simulink model "Hybrid_Beamforming"  (R2022b)
settings: Solver=FixedStepDiscrete  StartTime=0.0  StopTime=10  RelTol=1e-3
PreLoadFcn:
  | helperslexHybridBeamformingParam;
undefined symbols (not defined in the file or in its folder): paramHybridBF
libraries: dspmtrx3 x5, simulink x2, commrandsrc3 x1, phasedtxrxlib x1, commdigbbndam3 x1
CloseFcn:
  | clear paramHybridBF;
settings Model: FPTRunName=Active  ModifiedByFormat=The MathWorks Inc.  SimulationMode=accelerator  Creator=The MathWorks, Inc.  LastModifiedBy=The MathWorks Inc.
settings SolverCC: AlgebraicLoopSolver=TrustRegion  MaxZcPerStep=1
settings DataIOCC: LimitDataPoints=on  SaveFormat=Structure  SaveOutput=off  DSMLogging=off  SaveTime=off  ReturnWorkspaceOutputs=off
settings OptimizationCC: BlockReduction=off  ConditionallyExecuteInputs=off  DefaultParameterBehavior=Inlined  ExpressionDepthLimit=2147483647  LocalBlockOutputs=off  EfficientMapNaN2IntZero=off  LifeSpan=inf  SimCompilerOptimization=on
settings DebuggingCC: AlgebraicLoopMsg=error  UnderspecifiedInitializationDetection=Classic  MergeDetectMultiDrivingBlocksExec=none  SolverPrmCheckMsg=warning  MultiTaskDSMMsg=warning  MultiTaskCondExecSysMsg=none  SingleTaskRateTransMsg=error  IntegerOverflowMsg=none  ParameterPrecisionLossMsg=none  FcnCallInpInsideContextMsg=warning  UnconnectedInputMsg=warning  UnconnectedOutputMsg=warning  UnconnectedLineMsg=warning  AllowSymbolicDim=off  StateNameClashWarn=warning  PregeneratedLibrarySubsystemCodeDiagnostic=none  SFUnexpectedBacktrackingDiag=warning  SFNoUnconditionalDefaultTransitionDiag=warning  SFExecutionAtInitializationDiag=none  SFMachineParentedDataDiag=warning  ArithmeticOperatorsInVariantConditions=warning
settings HardwareCC: ProdBitPerPointer=32  ProdBitPerSizeT=32  ProdBitPerPtrDiffT=32  ProdLargestAtomicFloat=None  ProdIntDivRoundTo=Undefined  ProdEndianess=Unspecified  ProdWordSize=32  ProdHWDeviceType=ASIC/FPGA->ASIC/FPGA  TargetBitPerPointer=64  TargetBitPerSizeT=64  TargetBitPerPtrDiffT=64  TargetLongLongMode=on  TargetIntDivRoundTo=Zero  TargetEndianess=LittleEndian  TargetWordSize=64  TargetHWDeviceType=MATLAB Host  ProdEqTarget=off
settings ModelReferenceCC: EnableRefExpFcnMdlSchedulingChecks=on  PropagateSignalLabelsOutOfModel=off
settings SFSimCC: SimUseLocalCustomCode=off  CustomCodeUndefinedFunction=UseInterfaceOnly
settings RTWCC: DLArmComputeVersion=19.05
settings CodeAppCC: MaxIdLength=128
settings GRTTargetCC: TargetLangStandard=C89/C90 (ANSI)  CombineOutputUpdateFcns=off  GRTInterface=on
settings ConfigComp: CovMetricSettings=dw  CovSaveCumulativeToWorkspaceVar=on  CovSaveSingleToWorkspaceVar=on  CovExternalEMLEnable=off  CovSFcnEnable=off

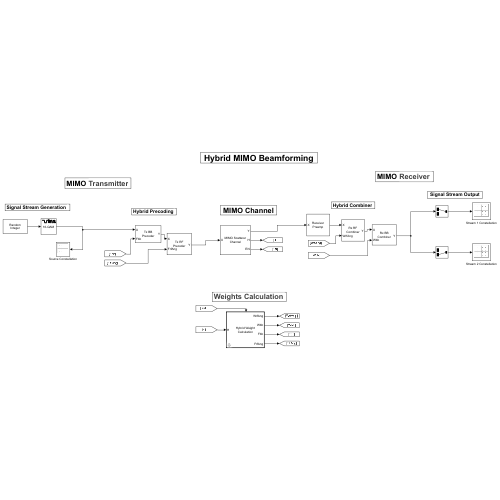
[thumbnail: Simulink's stored preview of the top-level diagram]
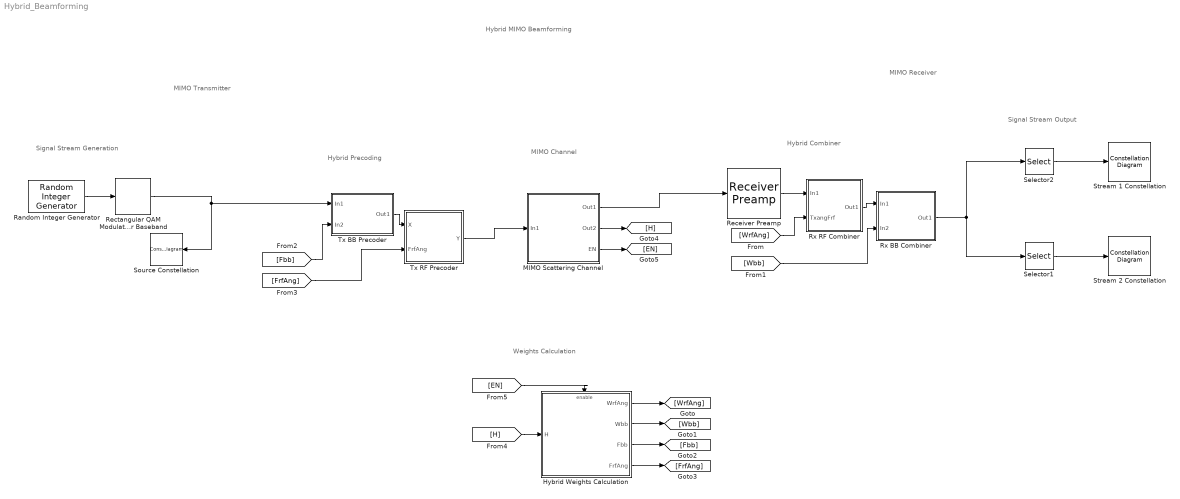
== system Hybrid_Beamforming ==
  note: Hybrid MIMO Beamforming
  note: Signal Stream Generation
  note: Hybrid Precoding
  note: MIMO Channel
  note: Signal Stream Output
  note: Hybrid Combiner
  note: Weights Calculation
  note: MIMO Transmitter
  note: MIMO Receiver
  Hybrid Weights Calculation : Subsystem  mask(Hybrid Beamforming Weights){Algorithm=QSHB, Ns=paramHybridBF.Ns, txpos=paramHybridBF.TxPos, NtRF=paramHybridBF.NtRF, rxpos=paramHybridBF.RxPos, NrRF=paramHybridBF.NrRF, txangF=paramHybridBF.TxAngF, rxangW=paramHybridBF.RxAngW, noisevar=1/paramHybridBF.SNR}
      mask prompts: Ns "Number of Data Streams"; txpos "Transmit Antenna Position"; NtRF "Number of Transmit RF Chain"; rxpos "Receive Antenna Position"; NrRF "Number of Receive RF Chain"; txangF "Transmit Direction Grid"; rxangW "Receive Direction Grid"; noisevar "Noise Power"
      mask help: Compute precoding and combining weights based on MIMO channel matrix
      mask init:
      | if strcmp(Algorithm,'QSHB')
      |     WSEL = 1;
      | else
      |     WSEL = 0;
      | end
      mask TypeOptions Algorithm: QSHB | HBPS
      mask Display:
      | disp('Hybrid Weight\nCalculation');
      | port_label('input',1,'H');
      | port_label('output',1,'WrfAng');
      | port_label('output',2,'Wbb');
      | port_label('output',3,'Fbb');
      | port_label('output',4,'FrfAng');
  MIMO Scattering Channel : Subsystem
      mask Display:
      | disp('MIMO Scatterer\nChannel');
      | port_label('input',1,'X');
      | port_label('output',1,'Y');
      | port_label('output',2,'H');
      | port_label('output',3,'EN');
  Random Integer Generator : commrandsrc3/Random Integer Generator  SetSize=paramHybridBF.M  SeedSource=Parameter  Seed=109  SampleTime=0.001  SamplesPerFrame=paramHybridBF.Ns  OutputDataType=double  SimulateUsing=Interpreted execution
  Receiver Preamp : phasedtxrxlib/Receiver Preamp  Gain=0  LossFactor=0  NoiseMethod=Noise power  NoiseFigure=0  ReferenceTemperature=290  SampleRateFromInputCheckbox=on  SampleRate=1e6  NoisePower=paramHybridBF.Ns/paramHybridBF.SNR  EnableInputPort=off  PhaseNoiseInputPort=off  SeedSource=Property  Seed=randi(65535,1)  SimulateUsing=Interpreted execution
  Rectangular QAM Modulator Baseband : commdigbbndam3/Rectangular QAM Modulator Baseband  M=paramHybridBF.M  InType=Integer  Enc=Gray  Mapping=[0:15]  PowType=Min. distance between symbols  MinDist=2/3  AvgPow=1  PeakPow=1  Ph=0  outDtype=double  outWordLen=16  outUDDataType=sfix(16)  outFracLenMode=Best precision  outFracLen=15  outDataTypeStr=double  outLastDataTypeStr=double
  Rx BB Combiner : Subsystem
      mask Display:
      | disp('Rx BB\nCombiner');
      | port_label('input',1,'X');
      | port_label('input',2,'Wbb');
      | port_label('output',1,'Y');
  Rx RF Combiner : Subsystem
      mask Display:
      | disp('Rx RF\nCombiner');
      | port_label('input',1,'X');
      | port_label('input',2,'WrfAng');
      | port_label('output',1,'Y');
  Selector1 : Selector  InputPortWidth=paramHybridBF.Ns  IndexOptions=Index vector (dialog)  Indices=2  OutputSizes=1
  Selector2 : Selector  InputPortWidth=paramHybridBF.Ns  IndexOptions=Index vector (dialog)  Indices=[1]  OutputSizes=1
  Source Constellation : ConstellationDiagram  WindowPosition=[298.000000,334.000000,438.000000,299.000000,]  ScopeFrameLocation=window  SymbolsToDisplaySource=Property  SymbolsToDisplay=paramHybridBF.NTxSym  ReferenceConstellation={[-10 -10]}  XLimits=[-2 2]  YLimits=[-2 2]  ShowReferenceConstellation=off  DefaultConfigurationName=comm.scopes.ConstellationDiagramBlockCfg
  Stream 1 Constellation : ConstellationDiagram  WindowPosition=[755.000000,331.000000,440.000000,303.000000,]  ScopeFrameLocation=window  SymbolsToDisplaySource=Property  SymbolsToDisplay=1000  ReferenceConstellation="{[-1+1i              -1+0.33333i              -1-0.33333i                    -1-1i              -0.33333+1i        -0.33333+0.33333i        -0.33333-0.33333i              -0.33333-1i               0.33333+1i         0.33333+0.33333i         0.33333-0.33333i               0.33333-1i                     1+1i               1+0.33333i               1-0.33333i                     1-1i]}"  XLimits=[-2 2]  YLimits=[-2 2]  DefaultConfigurationName=comm.scopes.ConstellationDiagramBlockCfg
  Stream 2 Constellation : ConstellationDiagram  WindowPosition=[788.000000,213.000000,485.000000,463.000000,]  ScopeFrameLocation=window  SymbolsToDisplaySource=Property  SymbolsToDisplay=1000  ReferenceConstellation="{[-1+1i              -1+0.33333i              -1-0.33333i                    -1-1i              -0.33333+1i        -0.33333+0.33333i        -0.33333-0.33333i              -0.33333-1i               0.33333+1i         0.33333+0.33333i         0.33333-0.33333i               0.33333-1i                     1+1i               1+0.33333i               1-0.33333i                     1-1i]}"  XLimits=[-2 2]  YLimits=[-2 2]  DefaultConfigurationName=comm.scopes.ConstellationDiagramBlockCfg
  Tx BB Precoder : Subsystem
      mask Display:
      | disp('Tx BB\nPrecoder');
      | port_label('input',1,'X');
      | port_label('Output',1,'Y');
      | port_label('Input',2,'Fbb');
  Tx RF Precoder : Subsystem
      mask Display:
      | disp('Tx RF\nPrecoder');
      | port_label('input',1,'X');
      | port_label('input',2,'FrfAng');
      | port_label('output',1,'Y');
  wires:
  Rx RF Combiner/1(Out1) -> Rx BB Combiner/1(In1)
  Rx BB Combiner/1(Out1) -> Selector2/1, Selector1/1
  Tx BB Precoder/1(Out1) -> Tx RF Precoder/1(X)
  Random Integer Generator/1 -> Rectangular QAM Modulator Baseband/1
  Rectangular QAM Modulator Baseband/1 -> Tx BB Precoder/1(In1), Source Constellation/1
  Selector1/1 -> Stream 2 Constellation/1
  Selector2/1 -> Stream 1 Constellation/1
  Tx RF Precoder/1(Y) -> MIMO Scattering Channel/1(In1)
  Hybrid Weights Calculation/1(WrfAng) -> [WrfAng]
  [WrfAng] -> Rx RF Combiner/2(TxangFrf)
  Hybrid Weights Calculation/2(Wbb) -> [Wbb]
  [Wbb] -> Rx BB Combiner/2(In2)
  Hybrid Weights Calculation/3(Fbb) -> [Fbb]
  [Fbb] -> Tx BB Precoder/2(In2)
  Hybrid Weights Calculation/4(FrfAng) -> [FrfAng]
  [FrfAng] -> Tx RF Precoder/2(FrfAng)
  MIMO Scattering Channel/2(Out2) -> [H]
  [H] -> Hybrid Weights Calculation/1(H)
  MIMO Scattering Channel/3(EN) -> [EN]
  [EN] -> Hybrid Weights Calculation/Enable
  MIMO Scattering Channel/1(Out1) -> Receiver Preamp/1
  Receiver Preamp/1 -> Rx RF Combiner/1(In1)

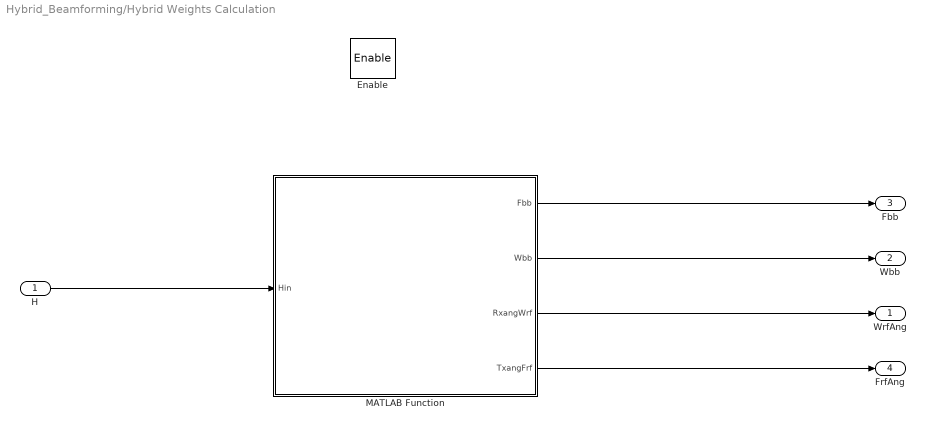
== system Hybrid_Beamforming/Hybrid Weights Calculation ==
  H : Inport
  Enable : EnablePort  PropagateVarSize=During execution
  MATLAB Function : MATLAB Function  TreatAsAtomicUnit=on
  WrfAng : Outport  VectorParamsAs1DForOutWhenUnconnected=off
  Wbb : Outport  Port=2  VectorParamsAs1DForOutWhenUnconnected=off
  Fbb : Outport  Port=3  VectorParamsAs1DForOutWhenUnconnected=off
  FrfAng : Outport  Port=4  VectorParamsAs1DForOutWhenUnconnected=off
  wires:
  H/1 -> MATLAB Function/1(Hin)
  MATLAB Function/1(Fbb) -> Fbb/1
  MATLAB Function/4(TxangFrf) -> FrfAng/1
  MATLAB Function/2(Wbb) -> Wbb/1
  MATLAB Function/3(RxangWrf) -> WrfAng/1

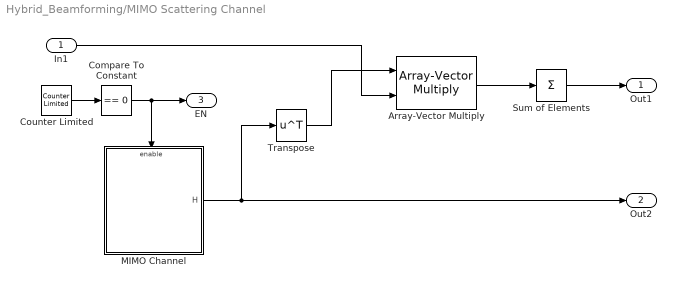
== system Hybrid_Beamforming/MIMO Scattering Channel ==
  In1 : Inport
  Array-Vector Multiply : dspmtrx3/Array-Vector Multiply  mode=Mute  saveAsFlag=0  Dimension=2  V_Source=Input port  V_VectFromMask=[0.5 0.25]  roundingMode=Floor  overflowMode=off  firstCoeffSignedness=Auto  firstCoeffDataTypeStr=Inherit: Same word length as input  firstCoeffMin=[]  firstCoeffMax=[]  firstCoeffLastDataTypeStr=Inherit: Same word length as input  prodOutputSignedness=Auto  accumSignedness=Auto  outputSignedness=Auto  outputDataTypeStr=Inherit: Same as product output  outputMin=[]  outputMax=[]  outputLastDataTypeStr=Inherit: Same as product output
  Compare To Constant : simulink/Logic and Bit Operations/Compare To Constant  relop===  const=0  OutDataTypeStr=boolean
  Counter Limited : simulink/Sources/Counter Limited  uplimit=paramHybridBF.NTxSym  tsamp=-1
  MIMO Channel : Subsystem
      mask Display:
      | disp('Channel')
      | port_label('output',1,'H')
      | port_label('input',1,'En')
  Sum of Elements : Sum  Inputs=+  CollapseMode=Specified dimension  CollapseDim=2
  Transpose : Math  Operator=transpose  SignedPower=on
  Out1 : Outport  VectorParamsAs1DForOutWhenUnconnected=off
  Out2 : Outport  Port=2  VectorParamsAs1DForOutWhenUnconnected=off
  EN : Outport  Port=3  VectorParamsAs1DForOutWhenUnconnected=off
  wires:
  Transpose/1 -> Array-Vector Multiply/1
  Compare To Constant/1 -> EN/1, MIMO Channel/Enable
  Counter Limited/1 -> Compare To Constant/1
  MIMO Channel/1(H) -> Transpose/1, Out2/1
  Array-Vector Multiply/1 -> Sum of Elements/1
  In1/1 -> Array-Vector Multiply/2
  Sum of Elements/1 -> Out1/1

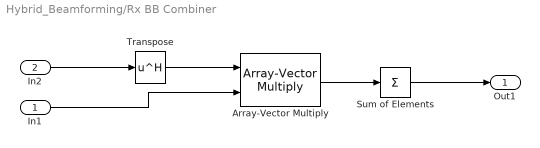
== system Hybrid_Beamforming/Rx BB Combiner ==
  In1 : Inport
  In2 : Inport  Port=2
  Array-Vector Multiply : dspmtrx3/Array-Vector Multiply  mode=Mute  saveAsFlag=0  Dimension=paramHybridBF.Ns  V_Source=Input port  V_VectFromMask=[0.5 0.25]  roundingMode=Floor  overflowMode=off  firstCoeffSignedness=Auto  firstCoeffDataTypeStr=Inherit: Same word length as input  firstCoeffMin=[]  firstCoeffMax=[]  firstCoeffLastDataTypeStr=Inherit: Same word length as input  prodOutputSignedness=Auto  accumSignedness=Auto  outputSignedness=Auto  outputDataTypeStr=Inherit: Same as product output  outputMin=[]  outputMax=[]  outputLastDataTypeStr=Inherit: Same as product output
  Sum of Elements : Sum  Inputs=+  CollapseMode=Specified dimension  CollapseDim=2
  Transpose : Math  Operator=hermitian  SignedPower=on
  Out1 : Outport  VectorParamsAs1DForOutWhenUnconnected=off
  wires:
  Array-Vector Multiply/1 -> Sum of Elements/1
  In2/1 -> Transpose/1
  Sum of Elements/1 -> Out1/1
  Transpose/1 -> Array-Vector Multiply/1
  In1/1 -> Array-Vector Multiply/2

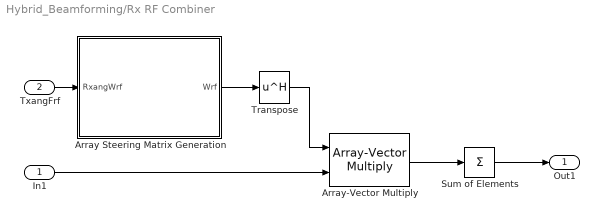
== system Hybrid_Beamforming/Rx RF Combiner ==
  In1 : Inport
  TxangFrf : Inport  Port=2
  Array Steering Matrix Generation : MATLAB Function  TreatAsAtomicUnit=on  mask(Steering Vector){RxPos=paramHybridBF.RxPos}
      mask prompts: RxPos "Receive Antenna Position"
      mask help: Compute array steering vector
  Array-Vector Multiply : dspmtrx3/Array-Vector Multiply  mode=Mute  saveAsFlag=0  Dimension=2  V_Source=Input port  V_VectFromMask=[0.5 0.25]  roundingMode=Floor  overflowMode=off  firstCoeffSignedness=Auto  firstCoeffDataTypeStr=Inherit: Same word length as input  firstCoeffMin=[]  firstCoeffMax=[]  firstCoeffLastDataTypeStr=Inherit: Same word length as input  prodOutputSignedness=Auto  accumSignedness=Auto  outputSignedness=Auto  outputDataTypeStr=Inherit: Same as product output  outputMin=[]  outputMax=[]  outputLastDataTypeStr=Inherit: Same as product output
  Sum of Elements : Sum  Inputs=+  CollapseMode=Specified dimension  CollapseDim=2
  Transpose : Math  Operator=hermitian  SignedPower=on
  Out1 : Outport  VectorParamsAs1DForOutWhenUnconnected=off
  wires:
  Array-Vector Multiply/1 -> Sum of Elements/1
  In1/1 -> Array-Vector Multiply/2
  Sum of Elements/1 -> Out1/1
  Transpose/1 -> Array-Vector Multiply/1
  TxangFrf/1 -> Array Steering Matrix Generation/1(RxangWrf)
  Array Steering Matrix Generation/1(Wrf) -> Transpose/1

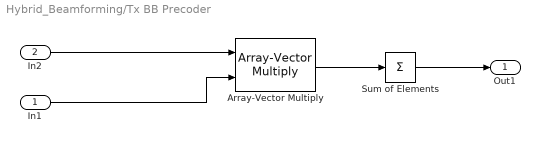
== system Hybrid_Beamforming/Tx BB Precoder ==
  In1 : Inport
  In2 : Inport  Port=2
  Array-Vector Multiply : dspmtrx3/Array-Vector Multiply  mode=Mute  saveAsFlag=0  Dimension=2  V_Source=Input port  V_VectFromMask=[0.5 0.25]  roundingMode=Floor  overflowMode=off  firstCoeffSignedness=Auto  firstCoeffDataTypeStr=Inherit: Same word length as input  firstCoeffMin=[]  firstCoeffMax=[]  firstCoeffLastDataTypeStr=Inherit: Same word length as input  prodOutputSignedness=Auto  accumSignedness=Auto  outputSignedness=Auto  outputDataTypeStr=Inherit: Same as product output  outputMin=[]  outputMax=[]  outputLastDataTypeStr=Inherit: Same as product output
  Sum of Elements : Sum  Inputs=+  CollapseMode=Specified dimension  CollapseDim=2
  Out1 : Outport  VectorParamsAs1DForOutWhenUnconnected=off
  wires:
  In2/1 -> Array-Vector Multiply/1
  In1/1 -> Array-Vector Multiply/2
  Array-Vector Multiply/1 -> Sum of Elements/1
  Sum of Elements/1 -> Out1/1

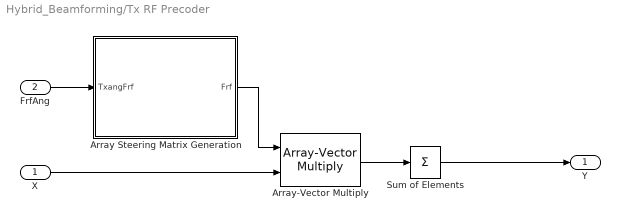
== system Hybrid_Beamforming/Tx RF Precoder ==
  X : Inport
  FrfAng : Inport  Port=2
  Array Steering Matrix Generation : MATLAB Function  TreatAsAtomicUnit=on  mask(Steering Vector){TxPos=paramHybridBF.TxPos}
      mask prompts: TxPos "Transmit Antenna Position"
      mask help: Compute array steering vector
  Array-Vector Multiply : dspmtrx3/Array-Vector Multiply  mode=Mute  saveAsFlag=0  Dimension=2  V_Source=Input port  V_VectFromMask=[0.5 0.25]  roundingMode=Floor  overflowMode=off  firstCoeffSignedness=Auto  firstCoeffDataTypeStr=Inherit: Same word length as input  firstCoeffMin=[]  firstCoeffMax=[]  firstCoeffLastDataTypeStr=Inherit: Same word length as input  prodOutputSignedness=Auto  accumSignedness=Auto  outputSignedness=Auto  outputDataTypeStr=Inherit: Same as product output  outputMin=[]  outputMax=[]  outputLastDataTypeStr=Inherit: Same as product output
  Sum of Elements : Sum  Inputs=+  CollapseMode=Specified dimension  CollapseDim=2
  Y : Outport  VectorParamsAs1DForOutWhenUnconnected=off
  wires:
  X/1 -> Array-Vector Multiply/2
  FrfAng/1 -> Array Steering Matrix Generation/1(TxangFrf)
  Array-Vector Multiply/1 -> Sum of Elements/1
  Sum of Elements/1 -> Y/1
  Array Steering Matrix Generation/1(Frf) -> Array-Vector Multiply/1

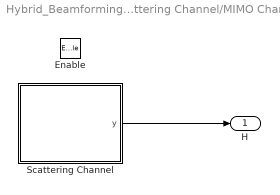
== system Hybrid_Beamforming/MIMO Scattering Channel/MIMO Channel ==
  Enable : EnablePort  PropagateVarSize=During execution
  "Scattering Channel " : MATLAB Function  TreatAsAtomicUnit=on  mask(MIMO Scattering Channel){txpos=paramHybridBF.TxPos, rxpos=paramHybridBF.RxPos}
      mask prompts: txpos "Tx Array Element Position"; rxpos "Rx Array Element Position"
      mask help: Create MIMO scattering channel matrix
  H : Outport  VectorParamsAs1DForOutWhenUnconnected=off
  wires:
  "Scattering Channel "/1(y) -> H/1

== matlab function Hybrid_Beamforming/Rx RF Combiner/Array Steering Matrix Generation ==
  data: RxangWrf input; Wrf output; RxPos parameter
function Wrf = fsteering_rx(RxangWrf,RxPos)
% Nr = size(RxPos,2);
% aa=ones(2,NrRF);
% arr=complex(zeros(Nr,NrRF));
% aa(:,1:NrRF)=RxangWrf(:,1:NrRF);
% 
% for i=1:NrRF
%     ang=aa(:,i);
%     arr(:,i)=steervec(RxPos,ang(:,1));
% end
% 
% Wrf = arr;

Wrf = steervec(RxPos,RxangWrf);

== matlab function Hybrid_Beamforming/Hybrid Weights Calculation/MATLAB Function ==
  data: Hin input; Fbb output; Wbb output; RxangWrf output; NtRF parameter; NrRF parameter; Ns parameter; txangF parameter; rxangW parameter; txpos parameter; rxpos parameter; noisevar parameter; Algorithm parameter; TxangFrf output
function [Fbb,Wbb, RxangWrf, TxangFrf] = hybridbfweights(Hin,NtRF, NrRF, Ns, txangF, rxangW, txpos, rxpos, noisevar, Algorithm)

if Algorithm==1  % QHCB
    H=Hin.';
    [~,~,v] = svd(H);
    [Nr,Nt] = size(H);
    Fopt = v(:,1:Ns);
    TxangFrf=zeros(2,NtRF);
    RxangWrf=zeros(2,NrRF);
    
    Frf = complex(zeros(Nt,NtRF));
    %Fbb = complex(zeros(NtRF,Ns));
    Fres = complex(zeros(Nt,Ns));  % Optimal matrix Fopt is genreated
    
    Adt = steervec(txpos,txangF);
    Ar = steervec(rxpos,rxangW);
    
    for m = 1:NtRF
        Psi = Adt'*Fres;
        [~,k] = max(diag(Psi*Psi'));
        Frf(:,m) = Adt(:,k);
        TxangFrf(:,m)=txangF(:,k); % save the angle for the steering vector which is in the space of Fopt
        Fbbtemp = (Frf(:,1:m)'*Frf(:,1:m))\Frf(:,1:m)'*Fopt;   %"\" is inverse of the matrix, that is the same as inv( )
        temp = Fopt-Frf(:,1:m)*Fbbtemp;
        Fres = temp/norm(temp,'fro');
    end
    
    Fbbtemp = sqrt(Ns)*Fbbtemp/norm(Frf*Fbbtemp,'fro');  % Calculate the basedband breamforming with giving the steering matrix
    Fbb = Fbbtemp(1:NtRF,1:Ns);
    
    Wmmse = ((Fbb'*Frf'*(H'*H)*Frf*Fbb+noisevar*Ns*eye(Ns))\Fbb'*Frf'*H')';     % Unconstrained Wopt for receiver
    Wrf = complex(zeros(Nr,NrRF));
    %Wbb = complex(zeros(NrRF,Ns));
    Wres = Wmmse;
    Ess = 1/Ns*eye(Ns);
    Eyy = H*Frf*Fbb*Ess*Fbb'*Frf'*H'+noisevar*eye(Nr);
    
    for m = 1:NrRF
        Psi = Ar'*Eyy*Wres;
        [~,k] = max(diag(Psi*Psi'));
        Wrf(:,m) = Ar(:,k);
        RxangWrf(:,m)=rxangW(:,k);  % save the angle for the steering vector which is in the space of Wopt
        Wbbtemp = (Wrf(:,1:m)'*Eyy*Wrf(:,1:m))\(Wrf(:,1:m)'*Eyy*Wmmse);
        temp = Wmmse-Wrf(:,1:m)*Wbbtemp;
        Wres = temp/norm(temp,'fro');
    end
    Wbb = Wbbtemp(1:NrRF,1:Ns);
    
else   % HBPS
    H=Hin.';
    [~,~,v] = svd(H);
    [Nr,Nt] = size(H);

    Fopt = v(:,1:Ns);

    At = steervec(txpos,txangF);  % Precalcualted array steering matrix.  Adt means array discrete Tx steering matrix 
    Ar = steervec(rxpos,rxangW);
    Psi= At'*Fopt;
    Ptxdiag=diag(Psi*Psi'); 
    %Ptxdiag1=diag(Psi*Psi'); 

    [~, inxa]=peaksearch(Ptxdiag,NtRF); 
    Frf=At(:,inxa);
    TxangFrf=txangF(:,inxa);

    Fbb = (Frf'*Frf)\Frf'*Fopt;   %Calculate the Fbb
    Fbb = sqrt(Ns)*Fbb/norm(Frf*Fbb,'fro');  % Calculate the basedband breamforming with giving the steering matrix 
                                             % Normalize Fbb

    %Wmmse = ((Fopt'*(H'*H)*Fopt+noisevar*Ns*eye(Ns))\Fopt'*H')';     % Unconstrained Wopt for receiver 
    Wmmse = (1/Ns*(Fbb'*Frf'*H')/(1/Ns*H*(Frf*(Fbb*Fbb')*Frf')*H'+noisevar*eye(Nr)))';
    Wres = Wmmse;
    Ess = 1/Ns*eye(Ns);
    Eyy = H*Frf*Fbb*Ess*Fbb'*Frf'*H'+noisevar*eye(Nr);

    Psirx=Ar'*Eyy*Wres;

    %Psirx=Ar'*Wres;

    Prxdiag1=diag(Psirx*Psirx');

    [~, inrxa]=peaksearch(Prxdiag1,NrRF); 
    Wrf=Ar(:,inrxa);
    RxangWrf=rxangW(:,inrxa);

    Wbb = (Wrf'*Eyy*Wrf)\(Wrf'*Eyy*Wmmse);
end

end

function [ymax, inx]= peaksearch(y, N)
%This function is to find the first N local maximums of value y and the
%index x 
% 10-1-2018

M=length(y); 
maxbuf=zeros(2,N);
b=0;
max=0;
dr=1;
inb1=1;
for i=1:M 
    a=y(i);
    if i>1 
        b=y(i-1);
    end
    max_mark=0;
    if a > b && dr == 1
        dr=1;
    elseif a <= b && dr == 1
        max=b;
        dr=-1;
        max_mark=1;
        inb1=i-1;
    elseif a > b && dr == -1
        dr=1;
    elseif  a<=b && dr == -1 
        dr=-1;
    end
    
    if max_mark==1
        for j=1:N
            if real(max) >= maxbuf(1,j) 
                for k=1:j
                    if j>1
                      maxbuf(:,j-1)=maxbuf(:,j);
                    end
                end
                maxbuf(1,j)=real(max);
                maxbuf(2,j)=inb1;
            end
        end          
    end
end
ymax=maxbuf(1,:);
inx=maxbuf(2,:);
end

== matlab function Hybrid_Beamforming/Tx RF Precoder/Array Steering Matrix Generation ==
  data: Frf output size=[paramHybridBF.Nt,paramHybridBF.NtRF]; TxangFrf input size=[2, paramHybridBF.NtRF]; TxPos parameter
function Frf = fsteering(TxangFrf,TxPos)

Frf = steervec(TxPos,TxangFrf);

== matlab function Hybrid_Beamforming/MIMO Scattering Channel/MIMO Channel/Scattering Channel  ==
  data: y output size=[paramHybridBF.Nt, paramHybridBF.Nr]; txpos parameter; rxpos parameter
function y  = fcn(txpos, rxpos)

rng(2019);           % Random Seed 
Ncl = 6;
Nray = 8;
Nscatter = Nray*Ncl;
angspread = 5;

% compute randomly placed scatterer clusters
txclang = [rand(1,Ncl)*60-30;rand(1,Ncl)*20-10];          % Azimuth from -30 degree to 30 degree.  Elevaton -10 degree to 10 degree.  
rxclang = [rand(1,Ncl)*120-60;rand(1,Ncl)*70-35];         % Make the cluster angle to Rx: azimuth range of -60 to 60 degree and the elevation range of -35 to 35



txang = zeros(2,Nscatter);
rxang = zeros(2,Nscatter);
% compute the rays within each cluster
for m = 1:Ncl
    txang(:,(m-1)*Nray+(1:Nray)) = randn(2,Nray)*angspread+diag(txclang(:,m))*ones(2,Nray);    %Calculate the scatter Tx angles arround each cluster 
    rxang(:,(m-1)*Nray+(1:Nray)) = randn(2,Nray)*angspread+diag(rxclang(:,m))*ones(2,Nray);    %Calculate the scatter Rx angles arround each cluster
end

greal=randn(1,Nscatter);
gimag=randn(1,Nscatter);
gg=(greal+1i*gimag)/sqrt(Nscatter);
y = scatteringchanmtx(txpos,rxpos,txang,rxang,gg);  % Calculate the scatter gain for every ray and normalized to 1 by dividing sqrt(Nscatter)
end
